simulink model "P2model"  (Simulink 9.1)
settings: Solver=VariableStepAuto  StartTime=0.0  StopTime=Tfin  FixedStep=dt  MaxStep=dtmax  RelTol=1e-3  EnableMultiTasking=on
values from neighbouring files (symbols this model uses):
  a = 1    [P2_1b.m]    (also in P2_laboratorio.m)
  A0 = 1    [P2_1b.m]    (also in P2_laboratorio.m)
  b = 1    [P2_1b.m]    (also in P2_laboratorio.m = 0.666666666667)
  f0 = 1/20    (= 0.05)    [P2_1b.m]    (also in P2_laboratorio.m)
  T = 0.2    [P2_1b.m]    (also in P2_laboratorio.m = 0.737)
settings Model: Creator=anonimo  LastModifiedBy=anonimo
settings SolverCC: ZeroCrossControl=EnableAll  AutoInsertRateTranBlk=on
settings DataIOCC: LimitDataPoints=on  SignalLoggingSaveFormat=ModelDataLogs  SaveTime=off
settings OptimizationCC: ExpressionDepthLimit=2147483647
settings DebuggingCC: SolverPrmCheckMsg=warning  FcnCallInpInsideContextMsg=warning  StateNameClashWarn=warning

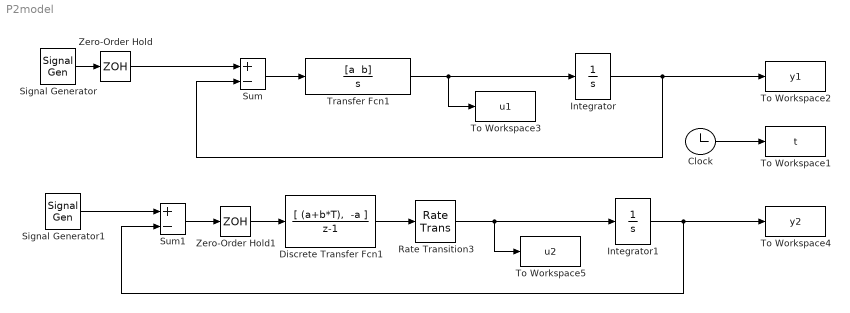
== system P2model ==
  Clock : Clock
  Discrete Transfer Fcn1 : DiscreteTransferFcn  Numerator="[ (a+b*T),  -a ]"  Denominator="[ 1,  -1]"  SampleTime=T
  Integrator : Integrator
  Integrator1 : Integrator
  Rate Transition3 : RateTransition  Deterministic=off
  Signal Generator : SignalGenerator  WaveForm=square  Amplitude=A0  Frequency=f0
  Signal Generator1 : SignalGenerator  WaveForm=square  Amplitude=A0  Frequency=f0
  Sum : Sum  Inputs=+-
  Sum1 : Sum  Inputs=+-
  To Workspace1 : ToWorkspace  VariableName=t  SampleTime=-1
  To Workspace2 : ToWorkspace  VariableName=y1  SampleTime=-1
  To Workspace3 : ToWorkspace  VariableName=u1  SampleTime=-1
  To Workspace4 : ToWorkspace  VariableName=y2  SampleTime=-1
  To Workspace5 : ToWorkspace  VariableName=u2  SampleTime=-1
  Transfer Fcn1 : TransferFcn  Numerator="[a  b]"  Denominator=[1 0]
  Zero-Order Hold : ZeroOrderHold  SampleTime=T
  Zero-Order Hold1 : ZeroOrderHold  SampleTime=T
  wires:
  Sum/1 -> Transfer Fcn1/1
  Integrator/1 -> Sum/2, To Workspace2/1
  Rate Transition3/1 -> To Workspace5/1, Integrator1/1
  Clock/1 -> To Workspace1/1
  Integrator1/1 -> Sum1/2, To Workspace4/1
  Signal Generator/1 -> Zero-Order Hold/1
  Transfer Fcn1/1 -> To Workspace3/1, Integrator/1
  Discrete Transfer Fcn1/1 -> Rate Transition3/1
  Zero-Order Hold1/1 -> Discrete Transfer Fcn1/1
  Sum1/1 -> Zero-Order Hold1/1
  Signal Generator1/1 -> Sum1/1
  Zero-Order Hold/1 -> Sum/1
